simulink model "vanguardlqg"  (Simulink 5.0)
settings: Solver=ode23s  StartTime=0.0  StopTime=10  RelTol=1e-3
values from neighbouring files (symbols this model uses):
  A = sqrt(ri*rf/(1-cos(phi)))*sin(phi)    [lambert.m]
  B = 2/re    (= 3.13571041087e-07)    [atmosphere.m]    (also in kepler.m = cos(e)-(pi/2-e)*sin(e))
  C = [dot(iprime,i),dot(iprime,j),dot(iprime,k);     dot(jprime,i),dot(jprime,j),dot(jprime,k);     dot(kprime,i),dot(kprime,j),dot(kprime,k)]    [Example2_2.m]    (also in orbit.m = eye(3))
  D = Qinf*S*CD    [accelclimb.m]    (also in airflight3dof.m; maneuver.m)
  K = liftddf(mach,CL,sweep,b^2/S)    [accelclimb.m]    (also in liftddf.m = S*K100+(1-S)*K0; maneuver.m)
  L = Qinf*S*CL    [accelclimb.m]    (also in aircoupled.m = q*S*b*(Clb*x(8)+0.5*b*(Clp*x(1)+Clr*x(3))/v); atmosphere.m = Vm/F; maneuver.m)
libraries: simulink x1
settings Model: BlockReductionOpt=off  BooleanDataType=off

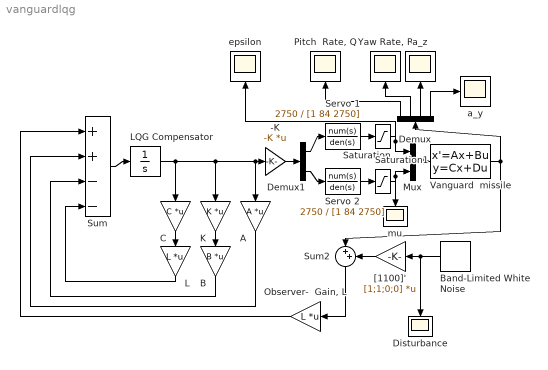
== system vanguardlqg ==
  " Servo 1" : TransferFcn  Numerator=2750  Denominator=[1 84 2750]
  -K : Gain  Gain=-K  Multiplication=Matrix(K*u)  SaturateOnIntegerOverflow=on
  A : Gain  Orientation=down  Gain=A  Multiplication=Matrix(K*u)  SaturateOnIntegerOverflow=on
  B : Gain  Orientation=down  Gain=B  Multiplication=Matrix(K*u)  SaturateOnIntegerOverflow=on
  Band-Limited White Noise : simulink/Sources/Band-Limited White Noise  Orientation=left  Cov=[1e-11]  Ts=0.1  seed=[23341]
  C : Gain  Orientation=down  Gain=C  Multiplication=Matrix(K*u)  SaturateOnIntegerOverflow=on
  Demux : Demux  Orientation=up
  Demux1 : Demux  Outputs=2
  Disturbance : Scope
      settings: Orientation=down  SaveName=d  DataFormat=Array
  K : Gain  Orientation=down  Gain=K  Multiplication=Matrix(K*u)  SaturateOnIntegerOverflow=on
  L : Gain  Orientation=down  Gain=L  Multiplication=Matrix(K*u)  SaturateOnIntegerOverflow=on
  LQG Compensator : Integrator
  Mux : Mux  Inputs=2
  "Observer-  Gain, L" : Gain  Orientation=left  Gain=L  Multiplication=Matrix(K*u)  SaturateOnIntegerOverflow=on
  "Pitch  Rate, Q" : Scope
      settings: Orientation=up  SaveName=Q  DataFormat=Array
  Saturation : Saturate  UpperLimit=0.01  LowerLimit=-0.01
  Saturation1 : Saturate  UpperLimit=0.1  LowerLimit=-0.1
  Servo 2 : TransferFcn  Numerator=2750  Denominator=[1 84 2750]
  Sum : Sum  Inputs=|++--  SaturateOnIntegerOverflow=on  InputSameDT=on
  Sum2 : Sum  Orientation=down  Inputs=|++  SaturateOnIntegerOverflow=on  InputSameDT=on
  Vanguard  missile : StateSpace  A=A  B=B  C=C  D=D  X0=[0;0;0;0;0.01;0.01]
  "Yaw Rate, R" : Scope
      settings: Orientation=up  SaveName=R  DataFormat=Array
  "[1100]'" : Gain  Orientation=left  Gain=[1;1;0;0]  Multiplication=Matrix(K*u)  SaturateOnIntegerOverflow=on
  a_y : Scope
      settings: SaveName=ay  DataFormat=Array
  a_z : Scope
      settings: Orientation=up  SaveName=az  DataFormat=Array
  epsilon : Scope
      settings: Orientation=up  SaveName=epsilon  DataFormat=Array
  mu : Scope
      settings: Orientation=down  SaveName=mu  DataFormat=Array
  wires:
  "Observer-  Gain, L"/1 -> Sum/1
  Sum/1 -> LQG Compensator/1
  C/1 -> L/1
  K/1 -> B/1
  L/1 -> Sum/4
  B/1 -> Sum/3
  A/1 -> Sum/2
  Sum2/1 -> "Observer-  Gain, L"/1
  LQG Compensator/1 -> C/1, K/1, -K/1, A/1
  Band-Limited White Noise/1 -> "[1100]'"/1, Disturbance/1
  "[1100]'"/1 -> Sum2/2
  Demux/2 -> "Yaw Rate, R"/1
  Demux/3 -> a_z/1
  Demux/4 -> a_y/1
  Vanguard  missile/1 -> Demux/1, Sum2/1
  -K/1 -> Demux1/1
  Demux1/1 -> " Servo 1"/1
  Demux1/2 -> Servo 2/1
  Mux/1 -> Vanguard  missile/1
  " Servo 1"/1 -> Saturation/1
  Servo 2/1 -> Saturation1/1
  Saturation/1 -> Mux/1, epsilon/1
  Saturation1/1 -> Mux/2, mu/1
  Demux/1 -> "Pitch  Rate, Q"/1
